simulink model "probnaSymulacja"  (R2017a)
settings: Solver=VariableStepAuto  StartTime=0.0  StopTime=40  MaxStep=0.01  MinStep=0.001  RelTol=1e-3
undefined symbols (not defined in the file or in its folder): A180, B180
settings Model: Creator=Szwank  LastModifiedBy=Szwank

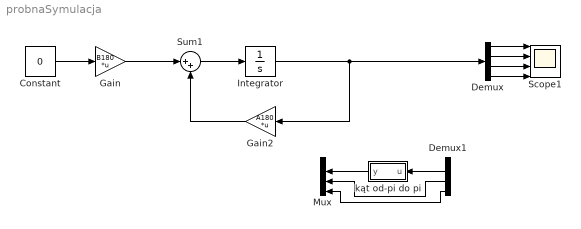
== system probnaSymulacja ==
  Constant : Constant  Value=0
  Demux : Demux
  Demux1 : Demux
  Gain : Gain  Gain=B180  Multiplication=Matrix(K*u)
  Gain2 : Gain  Gain=A180  Multiplication=Matrix(K*u)
  Integrator : Integrator  InitialCondition=[0 -pi 0 0]
  Mux : Mux
  Scope1 : Scope  NumInputPorts=4
  Sum1 : Sum  Inputs=|++
  kąt od-pi do pi : MATLAB Function  TreatAsAtomicUnit=on
  wires:
  Gain/1 -> Sum1/1
  Sum1/1 -> Integrator/1
  Gain2/1 -> Sum1/2
  Constant/1 -> Gain/1
  Integrator/1 -> Demux/1, Gain2/1
  Demux/1 -> Scope1/1
  Demux/2 -> Scope1/2
  Demux/3 -> Scope1/3
  Demux/4 -> Scope1/4
  Demux1/4 -> Mux/4
  kąt od-pi do pi/1(y) -> Mux/2
  Demux1/3 -> Mux/3
  Demux1/2 -> kąt od-pi do pi/1(u)

== matlab function probnaSymulacja/kąt od-pi do pi ==
  data: u input; y output
function y = fcn(u)

u=rem(u,2*pi);


if(u>0)
    if(u>pi)
        u=-pi+rem(u,pi);
    end
end

if(u<0)
    if(u<-pi)
        u=pi+rem(u,pi);
    end
end
y = u;
